simulink model "psbtransfohyst"  (Simulink 6.0)
settings: Solver=ode23tb  SolverMode=SingleTasking  StartTime=0.0  StopTime=0.2  FixedStep=50e-6  RelTol=1e-3
libraries: powerlib2 x11, powerlib_modelsV2 x1, simulink x1
settings Model: Creator=patrice  LastModifiedBy=batserve  ExtModeTrigMode=oneshot  ExtModeArmWhenConnect=off  ExtModeAutoUpdateStatusClock=off
settings DataIOCC: LimitDataPoints=off  SignalLoggingName=sigsOut
settings OptimizationCC: BlockReduction=off  BooleanDataType=off
settings DebuggingCC: AlgebraicLoopMsg=none  CheckExecutionContextPreStartOutputMsg=on  CheckExecutionContextRuntimeOutputMsg=on  SolverPrmCheckMsg=none
settings HardwareCC: TargetUnknown=on
settings RTWCC: TemplateMakefile=grt_unix.tmf

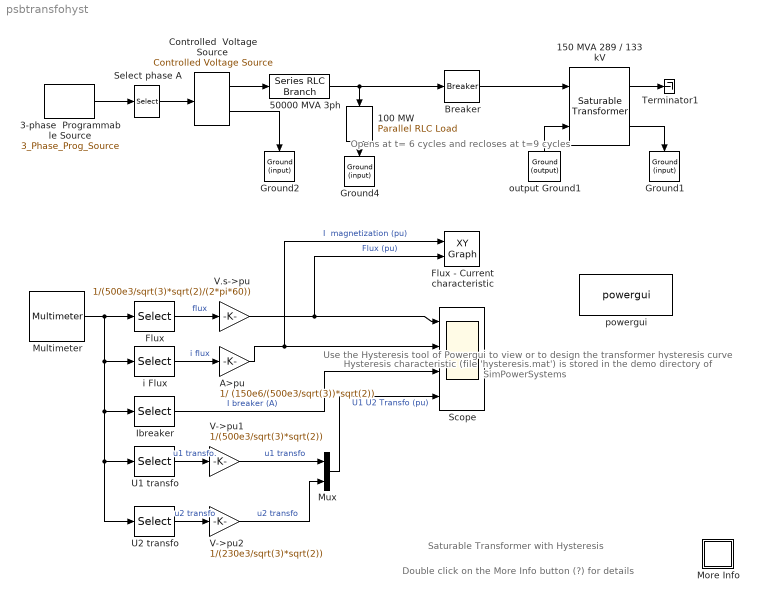
== system psbtransfohyst ==
  note: Saturable Transformer with Hysteresis
  note: Use the Hysteresis tool of Powergui to view
      | or to design the transformer hysteresis curve
  note: Hysteresis characteristic (file  'hysteresis.mat')
      | is stored in the demo directory of SimPowerSystems
  note: Opens  at t= 6 cycles
      | and recloses at t=9 cycles
  note: Double click on the More Info button (?) for details
  100 MW : powerlib2/Elements/Parallel RLC Load  Tag=PoWeRsYsTeMbLoCk  Orientation=down  a=500e3/sqrt(3)  b=60  c=100e6  d=0  e=0  mesure=None  PSBOutputType=1
  150 MVA 289 / 133 kV : powerlib2/Elements/Saturable Transformer  Tag=PoWeRsYsTeMbLoCk  a=[ 150e6 60 ]  b=[ 500e3/sqrt(3) 0.002 0.08 ]  c=[ 230e3/sqrt(3) 0.002 0.08]  w3check=off  d=[ 230e3/sqrt(3) 0.002 0.08]  e="[0 0;  0.0 1.1; 1.0  1.5]"  f=[200 0]  H=on  matfile='hysteresis'  Initialslope=+1  mesure=All measurements (V I Flux)  PSBOutputType=1111
  3-phase  Programmable Source : powerlib_modelsV2/Continuous/3_Phase_Prog_Source  Par_Vps_LLrms=[500e3*0.8 90 60]  VariationEntity=Amplitude  VariationType=Step  VariationStep=0.3  VariationRate=2  VariationMag=60  VariationFreq=1  Par_Timing_Variation=[0.05 1]  SinglePhase=off  Yampli=[1 0.8 1.2 1.0]  Xtime=[0 0.1 0.15 0.2]  HarmonicGeneration=off  Par_HarmoA_pu=[3 0.2 -25 0]  Par_HarmoB_pu=[2 0.15 35 2]  Par_Timing_Harmo="[0.05  1]"
  50000 MVA 3ph : powerlib2/Elements/Series RLC Branch  Tag=PoWeRsYsTeMbLoCk  a=500e3^2/5000e6/10  b=500e3^2/5000e6/(2*pi*60)  c=inf  mesure=Branch current  PSBOutputType=1
  A>pu : Gain  Gain=1/ (150e6/(500e3/sqrt(3))*sqrt(2))  SaturateOnIntegerOverflow=on
  Breaker : powerlib2/Elements/Breaker  Tag=PoWeRsYsTeMbLoCk  a=0.01  c=1  rs=1e7  cs=inf  times="[ 6/60  9/60]"  Ts=0  comext=off  mesure=None  PSBOutputType=1
  Controlled  Voltage Source : powerlib2/Electrical Sources/Controlled Voltage Source  Tag=PoWeRsYsTeMbLoCk  Description=source block  initsrc=on  srctyp=AC  iv=100  iph=0  ifreq=0  mesure=None  PSBOutputType=11
  Flux : Selector  InputPortWidth=5
  Flux - Current characteristic : simulink/Sinks/XY Graph  xmin=-0.05  xmax=0.05  ymin=-1.5  ymax=1.5  st=-1
  Ground1 : powerlib2/Connectors/Ground (input)  Tag=PoWeRsYsTeMbLoCk  Orientation=down
  Ground2 : powerlib2/Connectors/Ground (input)  Tag=PoWeRsYsTeMbLoCk  Orientation=down
  Ground4 : powerlib2/Connectors/Ground (input)  Tag=PoWeRsYsTeMbLoCk  Orientation=down
  Ibreaker : Selector  Elements=3  InputPortWidth=5
  More Info : Subsystem
      mask Display: disp('?')
  Multimeter : powerlib2/Measurements/Multimeter  Tag=PoWeRsYsTeMmEaSuReMeNt  PhasorSimulation=off  OutputType=Magnitude  sel=[8 7 4 1 2]  L=8  Gain=[1 1 1 1 1]  yselected={'Flux: 150 MVA 289 // 133 kV','Imag: 150 MVA 289 // 133 kV','Iw1: 150 MVA 289 // 133 kV','Uw1: 150 MVA 289 // 133 kV','Uw2: 150 MVA 289 // 133 kV'};  PSBOutputType=1  PSBequivalent=1  AxesSetting=[0,0.1,-100,100]  Display=0  SavedBlockNames=-11
  Mux : Mux  Inputs=2
  Scope : Scope  NumInputPorts=4
      settings: DeleteFcn=simscope BlockIsBeingDestroyed  PostSaveFcn=simscope Save  TimeRange=0.2  YMin=-2~-0.0238367~-1000~-2  YMax=2~0.0271003~2000~2  DataFormat=Array
  Select phase A : Selector  InputPortWidth=3
  Terminator1 : Terminator
  U1 transfo : Selector  Elements=4  InputPortWidth=5
  U2 transfo : Selector  Elements=5  InputPortWidth=5
  V->pu1 : Gain  Gain=1/(500e3/sqrt(3)*sqrt(2))  SaturateOnIntegerOverflow=on
  V->pu2 : Gain  Gain=1/(230e3/sqrt(3)*sqrt(2))  SaturateOnIntegerOverflow=on
  V.s->pu : Gain  Gain=1/(500e3/sqrt(3)*sqrt(2)/(2*pi*60))  SaturateOnIntegerOverflow=on
  i Flux : Selector  Elements=2  InputPortWidth=5
  output Ground1 : powerlib2/Connectors/Ground (output)  Tag=PoWeRsYsTeMbLoCk  Orientation=up  PSBOutputType=1
  powergui : powerlib2/powergui  Frange=[0:2:500]  Ylog=off  Xlog=on  save=off  variable=ZData  ZoomFFT=on  StartTime=0.0  cycles=1  DisplayStyle=off  fundamental=60  FreqAxis=off  MaxFrequency=1000  frequencyindice=1  frequencyindicesteady=1  RmsSteady=1  display=off  Ts=35e-6  methode=off  frequency=60  echomessages=off
  wires:
  50000 MVA 3ph/1 -> Breaker/1, 100 MW/1
  i Flux/1 -> A>pu/1  "i flux"
  Flux/1 -> V.s->pu/1  "flux"
  U1 transfo/1 -> V->pu1/1  "u1 transfo."
  3-phase  Programmable Source/1 -> Select phase A/1
  Select phase A/1 -> Controlled  Voltage Source/1
  Controlled  Voltage Source/2 -> Ground2/1
  U2 transfo/1 -> V->pu2/1  "u2 transfo"
  150 MVA 289 / 133 kV/2 -> Ground1/1
  Breaker/1 -> 150 MVA 289 / 133 kV/1
  V.s->pu/1 -> Flux - Current characteristic/2, Scope/1  "Flux (pu)"
  A>pu/1 -> Flux - Current characteristic/1, Scope/2  "I  magnetization (pu)"
  Controlled  Voltage Source/1 -> 50000 MVA 3ph/1
  Ibreaker/1 -> Scope/3  "I breaker (A)"
  Multimeter/1 -> Flux/1, i Flux/1, Ibreaker/1, U1 transfo/1, U2 transfo/1
  V->pu1/1 -> Mux/1  "u1 transfo"
  V->pu2/1 -> Mux/2  "u2 transfo"
  Mux/1 -> Scope/4  "U1 U2 Transfo (pu)"
  100 MW/1 -> Ground4/1
  output Ground1/1 -> 150 MVA 289 / 133 kV/2
  150 MVA 289 / 133 kV/1 -> Terminator1/1

== system psbtransfohyst/More Info ==
  note: S. Casoria (Hydro-Quebec) and P. Brunelle (TransEnergie)
  note: Demonstration
  note: Circuit Description
  note: This demonstration illustrates simulation of hystersis in a saturable transformer
  note: One phase of a three-phase transformer  is connected on a 500 kV network. The transformer is rated 500 kV/230 kV, 450 MVA (150 MVA per phase).
      | The flux-current saturation characteristic of the transformer is modelled with the hysteresis or with a simple  piecewise nonlinear characteristic.
      |
      | A programmable source is used to vary the internal voltage of the equivalent 500 kV network.
      | During the first 3 cycles source voltage is programmed at 0.8 pu. Then, at t = 3 cycles (0.05 s) voltage is increased to 1.1 pu.
      | In order to illustrate remanent flux and inrush current at transformer energization the circuit breaker which is initially closed
      | is first opened at t = 6 cycles (0.1 s),  then it is reclosed at t = 9 cycles (0.15 s).
      |
      | Initial flux in the transformer is set at zero and source phase angle is adjusted at 90 degrees so that flux remains symetrical around zero
      | when simulation is started.
      |
      | A Multimeter block and a Scope block are used to monitor waveforms of flux, magnetization current (not including the eddy currrents
      | which are modelled by the Rm resistance), voltages and current flowing into primary winding.
      | A X-Y Graph block is used to monitor the transformer operating point moving on the flux-current characteristic.
  note: Open the transformer menu and check that 'Simulate hysteresis' has been checked.
      | Using the 'Hysteresis design' tool of the powergui, load the hysteresis characteristic (load file 'hysteresis.mat').
      | Notice that flux and excitation current are displayed in pu. Using the 'Parameter units' popu menu, you can convert the pu units to SI units.
      | The saturation characteristics consists of two regions:
      |      1) The main hysteresis loop  : In this region there are 2 different flux values for a single current value.
      |      2) The saturated region defined by a simple line segment starting from the maximum point (Is,Fs) of the main loop.
      | The hysteresis loop is defined by the following 3 points marked by red dots on the main loop:
      |     [I=0; Remanent flux (Fr = 0.85pu)], [Coercive Current(Ic = 0.004 pu) ; F = 0] , [Saturation current (Is = 0.015 pu) ; Saturation flux (Fs = 1.2 pu)]
      |     plus the slope dF/dI at coercive current (F = 0).
      | Using the 'Zoom around hysteresis' checkbox and 'Display' button you can view the whole charactersitic or zoom on the hysteresis.
      |
      | Start the simulation and observe the following phenomena on the two scope blocks:
  note: Voltage and flux peak values are at 0.8 pu. Notice typical square wave of magnetization current.
      | As no remanent flux was specified, magnetization current and flux are symetrical. Flux travels on inner loops (inside the main loop).
  note: Voltage is 1.1 pu. Flux now reaches 1.1 pu and it travels on the main loop.
      | Current pulses appear on the magnetization current (2nd trace, I flux), indicating begining of saturation.
  note: At first zero crossing after the breaker opening order, current is interrupted and a flux of 0.83 pu stays trapped in the transformer core.
  note: The breaker is reclosed at t = 9 cycles, at a zero crossing of source voltage, producing an additional flux offset of approximatlely 1 pu.
      | The peak flux now reaches 1.85 pu, driving the transformer into the saturated region. Peak excitation current is 0.8 pu.
  note: 1) Simulation of saturation with hysteresis
  note: 2) Simulation of saturation with a piecewise nonlinear characteristic
  note: Open the transformer menu and deselect 'Simulate hysteresis'. The saturation will now be simulated by a piecewise nonlinear single-valued characteristic
      | defined by 7 points. Current/Flux pairs (in pu) are: [0 0;  0.0 0.85; 0.015 1.2;  0.03 1.35; 0.06 1.5; 0.09 1.56; 0.12 1.572].
      | The saturated region is the same, but the hysteresis loop is not simulated. Note that  this single valued characteristics still allows specifation
      | of a remanent flux of 0.85 pu (flux at zero magnetization current).
      | Start simulation and compare waveforms.
  note: From 0 to 0.05 sec. :
  note: From 0.05 sec. to 0.1 sec. :
  note: From 0.1 sec. to 0.15 sec. :
  note: From 0.15 sec. to 0.2 sec. :
